simulink model "astron_wb_fft_util"  (R2019a)
settings: Solver=VariableStepAuto  StartTime=0.0  StopTime=10.0  RelTol=1e-3
undefined symbols (not defined in the file or in its folder): FFT, Wideband_FFT_slim
libraries: xbsIndex_r4 x13
settings Model: Creator=talonm  LastModifiedBy=talonm

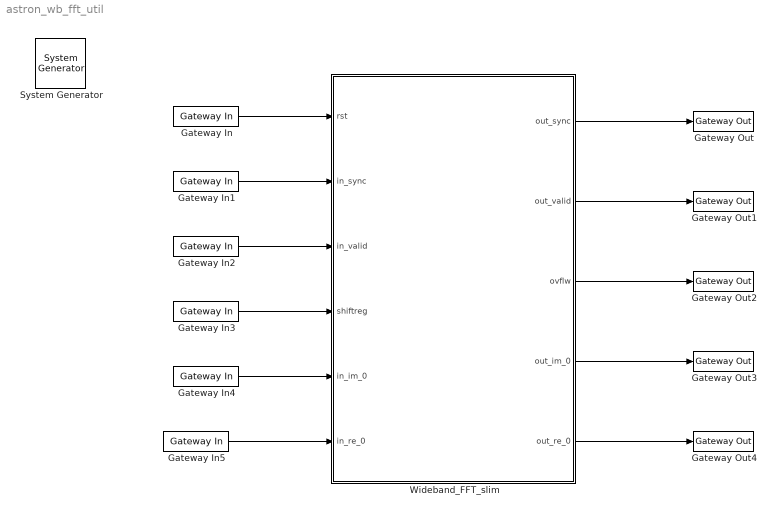
== system astron_wb_fft_util ==
  " System Generator" : xbsIndex_r4/ System Generator  Tag=genX  xilinxfamily=virtex7  part=xc7vx690t  speed=-1  package=ffg1927  synthesis_tool=Vivado  clock_wrapper=Clock Enables  directory=./netlist  proj_type=Vivado  Synth_file=Vivado Synthesis Defaults  Impl_file=Vivado Implementation Defaults  testbench=off  simulink_period=1  sysclk_period=10  dcm_input_clock_period=10  incr_netlist=off  trim_vbits=Everywhere in SubSystem  dbl_ovrd=According to Block Masks  core_generation=According to Block Masks  run_coregen=off  deprecated_control=off  eval_field=0  block_type=sysgen
  Gateway In : xbsIndex_r4/Gateway In  gui_display_data_type=Boolean  arith_type=Boolean  n_bits=16  bin_pt=14  preci_type=Single  exp_width=8  frac_width=24  rows=1  columns=1  quantization="Round  (unbiased: +/- Inf)"  overflow=Saturate  period=1  UseAsADC=off  ADCChannel='1'  interface=None  automatic_assignment=on  address_offset=hex2dec('00')  intf_name=''  intf_description=''  default_value=0  timing_constraint=None  locs_specified=off  LOCs={}  io_standard={}  inherit_from_input=off  hdl_port=on  dbl_ovrd=off  block_type=gatewayin
  Gateway In1 : xbsIndex_r4/Gateway In  gui_display_data_type=Boolean  arith_type=Boolean  n_bits=16  bin_pt=14  preci_type=Single  exp_width=8  frac_width=24  rows=1  columns=1  quantization="Round  (unbiased: +/- Inf)"  overflow=Saturate  period=1  UseAsADC=off  ADCChannel='1'  interface=None  automatic_assignment=on  address_offset=hex2dec('00')  intf_name=''  intf_description=''  default_value=0  timing_constraint=None  locs_specified=off  LOCs={}  io_standard={}  inherit_from_input=off  hdl_port=on  dbl_ovrd=off  block_type=gatewayin
  Gateway In2 : xbsIndex_r4/Gateway In  gui_display_data_type=Boolean  arith_type=Boolean  n_bits=16  bin_pt=14  preci_type=Single  exp_width=8  frac_width=24  rows=1  columns=1  quantization="Round  (unbiased: +/- Inf)"  overflow=Saturate  period=1  UseAsADC=off  ADCChannel='1'  interface=None  automatic_assignment=on  address_offset=hex2dec('00')  intf_name=''  intf_description=''  default_value=0  timing_constraint=None  locs_specified=off  LOCs={}  io_standard={}  inherit_from_input=off  hdl_port=on  dbl_ovrd=off  block_type=gatewayin
  Gateway In3 : xbsIndex_r4/Gateway In  gui_display_data_type=Fixed-point  arith_type=Unsigned  n_bits=10  bin_pt=0  preci_type=Single  exp_width=8  frac_width=24  rows=1  columns=1  quantization="Round  (unbiased: +/- Inf)"  overflow=Saturate  period=1  UseAsADC=off  ADCChannel='1'  interface=None  automatic_assignment=on  address_offset=hex2dec('00')  intf_name=''  intf_description=''  default_value=0  timing_constraint=None  locs_specified=off  LOCs={}  io_standard={}  inherit_from_input=off  hdl_port=on  dbl_ovrd=off  block_type=gatewayin
  Gateway In4 : xbsIndex_r4/Gateway In  gui_display_data_type=Fixed-point  arith_type="Signed  (2's comp)"  n_bits=18  bin_pt=17  preci_type=Single  exp_width=8  frac_width=24  rows=1  columns=1  quantization="Round  (unbiased: +/- Inf)"  overflow=Saturate  period=1  UseAsADC=off  ADCChannel='1'  interface=None  automatic_assignment=on  address_offset=hex2dec('00')  intf_name=''  intf_description=''  default_value=0  timing_constraint=None  locs_specified=off  LOCs={}  io_standard={}  inherit_from_input=off  hdl_port=on  dbl_ovrd=off  block_type=gatewayin
  Gateway In5 : xbsIndex_r4/Gateway In  gui_display_data_type=Fixed-point  arith_type="Signed  (2's comp)"  n_bits=18  bin_pt=17  preci_type=Single  exp_width=8  frac_width=24  rows=1  columns=1  quantization="Round  (unbiased: +/- Inf)"  overflow=Saturate  period=1  UseAsADC=off  ADCChannel='1'  interface=None  automatic_assignment=on  address_offset=hex2dec('00')  intf_name=''  intf_description=''  default_value=0  timing_constraint=None  locs_specified=off  LOCs={}  io_standard={}  inherit_from_input=off  hdl_port=on  dbl_ovrd=off  block_type=gatewayin
  Gateway Out{,1..4} (5 alike) : xbsIndex_r4/Gateway Out  inherit_from_input=off  hdl_port=on  rows=1  columns=1  UseAsDAC=off  DACChannel='1'  interface=None  automatic_assignment=on  address_offset=hex2dec('00')  intf_name=''  intf_description=''  timing_constraint=None  locs_specified=off  LOCs={}  io_standard={}  block_type=gatewayout
  Wideband_FFT_slim : Subsystem  AncestorBlock=FFT/Wideband_FFT_slim  mask{use_separate=on, use_fft_shift=off, use_reorder=on, nof_chan=0, wb_factor=1, twiddle_offset=0, nof_points=8192, xtra_dat_sigs=off, in_dat_w=18, out_dat_w=18, out_gain_w=0, stage_dat_w=18, guard_enable=off, guard_w=2, representation="SIGNED", use_round="ROUND", ovflw_behav="WRAP", use_dsp="YES", use_variant="4DSP", technology=0, ram_primitive="auto", fifo_primitive="auto"}
      mask prompts: use_separate "Separate complex in/out ports?"; use_fft_shift "Reorderder frequencies"; use_reorder "Bit reverse output"; nof_chan "Nof channels (time mux inputs)"; wb_factor "Wideband factor"; twiddle_offset "Twiddle offsets"; nof_points "Number of points"; xtra_dat_sigs "Extra control signals"; in_dat_w "Input data width"; out_dat_w "Ouput data width"; out_gain_w "Output gain width"; stage_dat_w "Stage data width"; guard_enable "Guard enable"; guard_w "Guard bit width"; representation "Data Representation"; use_round "Rounding Behaviour"; ovflw_behav "Overflow Behaviour"; use_dsp "Use DSP for Cmults"; use_variant "Cmult options"; technology "Vendor (0-Xilinx, 1-Intel)"; ram_primitive "Ram Primitive"; fifo_primitive "Fifo Primitive"
      mask init:
      | Simulink.Block.eval([gcb, '/wb_fft_slim']);
      | 
      | wb_slim_subsys2bb_knit();
      mask Callback use_separate:
      | % Control parameter visiblity
      | 
      | % Get the value of the Enable Bias checkbox
      | % unchecked = 'off'
      | % checked = 'on'
      | enab = get_param(gcb,'use_separate');
      | 
      | % Set the 'MaskVisibilities' property for each parameters
      | if strcmp(enab,'on')
      |     set_param(gcb,'use_reorder','on');
      |     set_param(gcb,'use_fft_shift','off');
      |     set_param(gcb,'MaskEnables',{'on','off','off','on','on','on','on','on','on','on','on','on','on','on','on','on','on','on','on','on','on','on'});
      | else
      |     set_param(gcb,'MaskEnables',{'on','on','on','on','on','on','on','on','on','on','on','on','on','on','on','on','on','on','on','on','on','on'});
      | end
      mask Callback use_fft_shift:
      | % Control parameter visiblity
      | 
      | % Get the value of the Enable Bias checkbox
      | % unchecked = 'off'
      | % checked = 'on'
      | enab = get_param(gcb,'use_fft_shift');
      | 
      | % Set the 'MaskVisibilities' property for each parameters
      | if strcmp(enab,'on')
      |     set_param(gcb,'use_reorder','on');
      |     set_param(gcb,'MaskEnables',{'on','on','off','on','on','on','on','on','on','on','on','on','on','on','on','on','on','on','on','on','on','on'});
      | else
      |     set_param(gcb,'MaskEnables',{'on','on','on','on','on','on','on','on','on','on','on','on','on','on','on','on','on','on','on','on','on','on'});
      | end
      mask Callback guard_enable:
      | % Control parameter visiblity
      | 
      | % Get the value of the Enable Bias checkbox
      | % unchecked = 'off'
      | % checked = 'on'
      | enab = get_param(gcb,'guard_enable');
      | 
      | % Set the 'MaskVisibilities' property for each parameters
      | if strcmp(enab,'on')
      |     set_param(gcb,'MaskVisibilities',{'on','on','on','on','on','on','on','on','on','on','on','on','on','on','on','on','on','on','on','on','on','on'});
      | else
      |     set_param(gcb,'MaskVisibilities',{'on','on','on','on','on','on','on','on','on','on','on','on','on','off','on','on','on','on','on','on','on','on'});
      | end
      mask TypeOptions representation: "SIGNED" | "UNSIGNED"
      mask TypeOptions use_round: "ROUND" | "TRUNCTATE"
      mask TypeOptions ovflw_behav: "WRAP" | "SATURATE"
      mask TypeOptions use_dsp: "YES" | "NO"
      mask TypeOptions use_variant: "4DSP" | "3DSP"
      mask TypeOptions technology: 0 | 1
      mask TypeOptions ram_primitive: "auto" | "block" | "distributed" | "ultra"
      mask TypeOptions fifo_primitive: "auto" | "block" | "distributed" | "ultra"
      mask DialogControl fft_params Prompt: FFT Parameters
      mask DialogControl data_params Prompt: Data Parameters
      mask DialogControl synth_imp Prompt: FPGA Synth/Imp
  wires:
  Gateway In/1 -> Wideband_FFT_slim/1(rst)
  Gateway In1/1 -> Wideband_FFT_slim/2(in_sync)
  Gateway In2/1 -> Wideband_FFT_slim/3(in_valid)
  Gateway In3/1 -> Wideband_FFT_slim/4(shiftreg)
  Gateway In4/1 -> Wideband_FFT_slim/5(in_im_0)
  Gateway In5/1 -> Wideband_FFT_slim/6(in_re_0)
  Wideband_FFT_slim/1(out_sync) -> Gateway Out/1
  Wideband_FFT_slim/2(out_valid) -> Gateway Out1/1
  Wideband_FFT_slim/3(ovflw) -> Gateway Out2/1
  Wideband_FFT_slim/4(out_im_0) -> Gateway Out3/1
  Wideband_FFT_slim/5(out_re_0) -> Gateway Out4/1

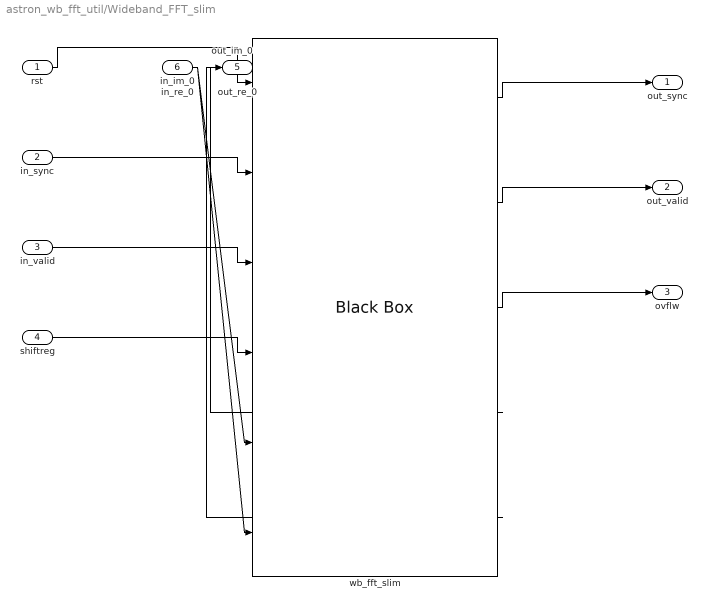
== system astron_wb_fft_util/Wideband_FFT_slim ==
  rst : Inport
  in_sync : Inport  Port=2
  in_valid : Inport  Port=3
  shiftreg : Inport  Port=4
  in_im_0 : Inport  Port=5
  in_re_0 : Inport  Port=6
  wb_fft_slim : xbsIndex_r4/Black Box  init_code=wideband_fft_slim_top_config  sim_method=ISE Simulator  verbose=off  block_type=blackbox2
  out_sync : Outport
  out_valid : Outport  Port=2
  ovflw : Outport  Port=3
  out_im_0 : Outport  Port=4
  out_re_0 : Outport  Port=5
  wires:
  rst/1 -> wb_fft_slim/1
  in_sync/1 -> wb_fft_slim/2
  wb_fft_slim/1 -> out_sync/1
  in_valid/1 -> wb_fft_slim/3
  wb_fft_slim/2 -> out_valid/1
  shiftreg/1 -> wb_fft_slim/4
  wb_fft_slim/3 -> ovflw/1
  in_im_0/1 -> wb_fft_slim/5
  in_re_0/1 -> wb_fft_slim/6
  wb_fft_slim/4 -> out_im_0/1
  wb_fft_slim/5 -> out_re_0/1
